simulink model "Deployed_On_CPU2"  (R2020a)
settings: Solver=ode4  StartTime=0.0  StopTime=Inf  FixedStep=0.01  RelTol=1e-3  EnableMultiTasking=on
undefined symbols (not defined in the file): C28x, CPU1, CPU2
libraries: c280xlib x47, dspobslib x27, simulink x20, c2837xDlib x1
(part 3 of 3)

== system Deployed_On_CPU2/Subsystem3/Pressure Sensor/Data acquisition/Subsystem/Delay 1ms10 ==
  function : TriggerPort  TriggerType=function-call  VariantControl=Variant
  System Outputs : Subsystem  mask(System Outputs){ShowInLibBrowser=0}
      mask prompts: ShowInLibBrowser "Simulink:masks:CustCodeMaskParam1_MP"
      settings: CopyFcn=cccopyfcn(gcb)  OpenFcn=ccopenfcn('System Outputs Function')
      mask Help: eval('feval(''rtwprivate'',''rtwhelpview'',''rtw_sys_outputs_block'')');
      mask Display: disp('System\nOutputs');

== system Deployed_On_CPU2/Subsystem3/Pressure Sensor/Data acquisition/Subsystem/Delay 1ms11 ==
  function : TriggerPort  TriggerType=function-call  VariantControl=Variant
  System Outputs : Subsystem  mask(System Outputs){ShowInLibBrowser=0}
      mask prompts: ShowInLibBrowser "Simulink:masks:CustCodeMaskParam1_MP"
      settings: CopyFcn=cccopyfcn(gcb)  OpenFcn=ccopenfcn('System Outputs Function')
      mask Help: eval('feval(''rtwprivate'',''rtwhelpview'',''rtw_sys_outputs_block'')');
      mask Display: disp('System\nOutputs');

== system Deployed_On_CPU2/Subsystem3/Pressure Sensor/Data acquisition/Subsystem/Delay 1ms12 ==
  function : TriggerPort  TriggerType=function-call  VariantControl=Variant
  System Outputs : Subsystem  mask(System Outputs){ShowInLibBrowser=0}
      mask prompts: ShowInLibBrowser "Simulink:masks:CustCodeMaskParam1_MP"
      settings: CopyFcn=cccopyfcn(gcb)  OpenFcn=ccopenfcn('System Outputs Function')
      mask Help: eval('feval(''rtwprivate'',''rtwhelpview'',''rtw_sys_outputs_block'')');
      mask Display: disp('System\nOutputs');

== system Deployed_On_CPU2/Subsystem3/Pressure Sensor/Data acquisition/Subsystem/Delay 1ms13 ==
  function : TriggerPort  TriggerType=function-call  VariantControl=Variant
  System Outputs : Subsystem  mask(System Outputs){ShowInLibBrowser=0}
      mask prompts: ShowInLibBrowser "Simulink:masks:CustCodeMaskParam1_MP"
      settings: CopyFcn=cccopyfcn(gcb)  OpenFcn=ccopenfcn('System Outputs Function')
      mask Help: eval('feval(''rtwprivate'',''rtwhelpview'',''rtw_sys_outputs_block'')');
      mask Display: disp('System\nOutputs');

== system Deployed_On_CPU2/Subsystem3/Pressure Sensor/Data acquisition/Subsystem/Delay 1ms2 ==
  function : TriggerPort  TriggerType=function-call  VariantControl=Variant
  System Outputs : Subsystem  mask(System Outputs){ShowInLibBrowser=0}
      mask prompts: ShowInLibBrowser "Simulink:masks:CustCodeMaskParam1_MP"
      settings: CopyFcn=cccopyfcn(gcb)  OpenFcn=ccopenfcn('System Outputs Function')
      mask Help: eval('feval(''rtwprivate'',''rtwhelpview'',''rtw_sys_outputs_block'')');
      mask Display: disp('System\nOutputs');

== system Deployed_On_CPU2/Subsystem3/Pressure Sensor/Data acquisition/Subsystem/Delay 1ms3 ==
  function : TriggerPort  TriggerType=function-call  VariantControl=Variant
  System Outputs : Subsystem  mask(System Outputs){ShowInLibBrowser=0}
      mask prompts: ShowInLibBrowser "Simulink:masks:CustCodeMaskParam1_MP"
      settings: CopyFcn=cccopyfcn(gcb)  OpenFcn=ccopenfcn('System Outputs Function')
      mask Help: eval('feval(''rtwprivate'',''rtwhelpview'',''rtw_sys_outputs_block'')');
      mask Display: disp('System\nOutputs');

== system Deployed_On_CPU2/Subsystem3/Pressure Sensor/Data acquisition/Subsystem/Delay 1ms4 ==
  function : TriggerPort  TriggerType=function-call  VariantControl=Variant
  System Outputs : Subsystem  mask(System Outputs){ShowInLibBrowser=0}
      mask prompts: ShowInLibBrowser "Simulink:masks:CustCodeMaskParam1_MP"
      settings: CopyFcn=cccopyfcn(gcb)  OpenFcn=ccopenfcn('System Outputs Function')
      mask Help: eval('feval(''rtwprivate'',''rtwhelpview'',''rtw_sys_outputs_block'')');
      mask Display: disp('System\nOutputs');

== system Deployed_On_CPU2/Subsystem3/Pressure Sensor/Data acquisition/Subsystem/Delay 1ms5 ==
  function : TriggerPort  TriggerType=function-call  VariantControl=Variant
  System Outputs : Subsystem  mask(System Outputs){ShowInLibBrowser=0}
      mask prompts: ShowInLibBrowser "Simulink:masks:CustCodeMaskParam1_MP"
      settings: CopyFcn=cccopyfcn(gcb)  OpenFcn=ccopenfcn('System Outputs Function')
      mask Help: eval('feval(''rtwprivate'',''rtwhelpview'',''rtw_sys_outputs_block'')');
      mask Display: disp('System\nOutputs');

== system Deployed_On_CPU2/Subsystem3/Pressure Sensor/Data acquisition/Subsystem/Delay 1ms6 ==
  function : TriggerPort  TriggerType=function-call  VariantControl=Variant
  System Outputs : Subsystem  mask(System Outputs){ShowInLibBrowser=0}
      mask prompts: ShowInLibBrowser "Simulink:masks:CustCodeMaskParam1_MP"
      settings: CopyFcn=cccopyfcn(gcb)  OpenFcn=ccopenfcn('System Outputs Function')
      mask Help: eval('feval(''rtwprivate'',''rtwhelpview'',''rtw_sys_outputs_block'')');
      mask Display: disp('System\nOutputs');

== system Deployed_On_CPU2/Subsystem3/Pressure Sensor/Data acquisition/Subsystem/Delay 1ms7 ==
  function : TriggerPort  TriggerType=function-call  VariantControl=Variant
  System Outputs : Subsystem  mask(System Outputs){ShowInLibBrowser=0}
      mask prompts: ShowInLibBrowser "Simulink:masks:CustCodeMaskParam1_MP"
      settings: CopyFcn=cccopyfcn(gcb)  OpenFcn=ccopenfcn('System Outputs Function')
      mask Help: eval('feval(''rtwprivate'',''rtwhelpview'',''rtw_sys_outputs_block'')');
      mask Display: disp('System\nOutputs');

== system Deployed_On_CPU2/Subsystem3/Pressure Sensor/Data acquisition/Subsystem/Delay 1ms8 ==
  function : TriggerPort  TriggerType=function-call  VariantControl=Variant
  System Outputs : Subsystem  mask(System Outputs){ShowInLibBrowser=0}
      mask prompts: ShowInLibBrowser "Simulink:masks:CustCodeMaskParam1_MP"
      settings: CopyFcn=cccopyfcn(gcb)  OpenFcn=ccopenfcn('System Outputs Function')
      mask Help: eval('feval(''rtwprivate'',''rtwhelpview'',''rtw_sys_outputs_block'')');
      mask Display: disp('System\nOutputs');

== system Deployed_On_CPU2/Subsystem3/Pressure Sensor/Data acquisition/Subsystem/Delay 1ms9 ==
  function : TriggerPort  TriggerType=function-call  VariantControl=Variant
  System Outputs : Subsystem  mask(System Outputs){ShowInLibBrowser=0}
      mask prompts: ShowInLibBrowser "Simulink:masks:CustCodeMaskParam1_MP"
      settings: CopyFcn=cccopyfcn(gcb)  OpenFcn=ccopenfcn('System Outputs Function')
      mask Help: eval('feval(''rtwprivate'',''rtwhelpview'',''rtw_sys_outputs_block'')');
      mask Display: disp('System\nOutputs');

== system Deployed_On_CPU2/Subsystem3/Pressure Sensor/Data acquisition/Subsystem/Read 6 bytes2 ==
  function : TriggerPort  TriggerType=function-call  VariantControl=Variant
  Add : Sum
  Data Type Conversion : DataTypeConversion  OutDataTypeStr=int16  ConvertRealWorld=Stored Integer (SI)
  Demux : Demux  Outputs=2
  Gain : Gain  Gain=256
  I2C Receive1 : c280xlib/I2C Receive  Priority=10  selectModule=I2C_A  addrFormat=7-Bit addressing  saSource=Specify via dialog  SAR=hex2dec('76')  bitCount=8  dataLength=2  initValue=0  NACK=off  STP=on  STR=on  sampleTime=-1  dataType=uint8
      settings: SourceProductBaseCode=TIC2000
  Terminator1 : Terminator
  Out1 : Outport
  wires:
  I2C Receive1/2 -> Terminator1/1
  I2C Receive1/1 -> Data Type Conversion/1
  Data Type Conversion/1 -> Demux/1
  Demux/1 -> Gain/1
  Demux/2 -> Add/2
  Gain/1 -> Add/1
  Add/1 -> Out1/1

== system Deployed_On_CPU2/Subsystem3/Pressure Sensor/Data acquisition/Subsystem/Read 6 bytes3 ==
  function : TriggerPort  TriggerType=function-call  VariantControl=Variant
  Add : Sum
  Data Type Conversion : DataTypeConversion  OutDataTypeStr=int16  ConvertRealWorld=Stored Integer (SI)
  Demux : Demux  Outputs=2
  Gain : Gain  Gain=256
  I2C Receive1 : c280xlib/I2C Receive  Priority=10  selectModule=I2C_A  addrFormat=7-Bit addressing  saSource=Specify via dialog  SAR=hex2dec('76')  bitCount=8  dataLength=2  initValue=0  NACK=off  STP=on  STR=on  sampleTime=-1  dataType=uint8
      settings: SourceProductBaseCode=TIC2000
  Terminator1 : Terminator
  Out1 : Outport
  wires:
  I2C Receive1/2 -> Terminator1/1
  I2C Receive1/1 -> Data Type Conversion/1
  Data Type Conversion/1 -> Demux/1
  Demux/1 -> Gain/1
  Add/1 -> Out1/1
  Gain/1 -> Add/1
  Demux/2 -> Add/2

== system Deployed_On_CPU2/Subsystem3/Pressure Sensor/Data acquisition/Subsystem/Read 6 bytes4 ==
  function : TriggerPort  TriggerType=function-call  VariantControl=Variant
  Add : Sum
  Data Type Conversion : DataTypeConversion  OutDataTypeStr=int16  ConvertRealWorld=Stored Integer (SI)
  Demux : Demux  Outputs=2
  Gain : Gain  Gain=256
  I2C Receive1 : c280xlib/I2C Receive  Priority=10  selectModule=I2C_A  addrFormat=7-Bit addressing  saSource=Specify via dialog  SAR=hex2dec('76')  bitCount=8  dataLength=2  initValue=0  NACK=off  STP=on  STR=on  sampleTime=-1  dataType=uint8
      settings: SourceProductBaseCode=TIC2000
  Terminator1 : Terminator
  Out1 : Outport
  wires:
  I2C Receive1/2 -> Terminator1/1
  I2C Receive1/1 -> Data Type Conversion/1
  Data Type Conversion/1 -> Demux/1
  Demux/1 -> Gain/1
  Add/1 -> Out1/1
  Gain/1 -> Add/1
  Demux/2 -> Add/2

== system Deployed_On_CPU2/Subsystem3/Pressure Sensor/Data acquisition/Subsystem/Read 6 bytes5 ==
  function : TriggerPort  TriggerType=function-call  VariantControl=Variant
  Add : Sum
  Data Type Conversion : DataTypeConversion  OutDataTypeStr=int16  ConvertRealWorld=Stored Integer (SI)
  Demux : Demux  Outputs=2
  Gain : Gain  Gain=256
  I2C Receive1 : c280xlib/I2C Receive  Priority=10  selectModule=I2C_A  addrFormat=7-Bit addressing  saSource=Specify via dialog  SAR=hex2dec('76')  bitCount=8  dataLength=2  initValue=0  NACK=off  STP=on  STR=on  sampleTime=-1  dataType=uint8
      settings: SourceProductBaseCode=TIC2000
  Terminator1 : Terminator
  Out1 : Outport
  wires:
  I2C Receive1/2 -> Terminator1/1
  I2C Receive1/1 -> Data Type Conversion/1
  Data Type Conversion/1 -> Demux/1
  Demux/1 -> Gain/1
  Add/1 -> Out1/1
  Gain/1 -> Add/1
  Demux/2 -> Add/2

== system Deployed_On_CPU2/Subsystem3/Pressure Sensor/Data acquisition/Subsystem/Read 6 bytes6 ==
  function : TriggerPort  TriggerType=function-call  VariantControl=Variant
  Add : Sum
  Data Type Conversion : DataTypeConversion  OutDataTypeStr=int16  ConvertRealWorld=Stored Integer (SI)
  Demux : Demux  Outputs=2
  Gain : Gain  Gain=256
  I2C Receive1 : c280xlib/I2C Receive  Priority=10  selectModule=I2C_A  addrFormat=7-Bit addressing  saSource=Specify via dialog  SAR=hex2dec('76')  bitCount=8  dataLength=2  initValue=0  NACK=off  STP=on  STR=on  sampleTime=-1  dataType=uint8
      settings: SourceProductBaseCode=TIC2000
  Terminator1 : Terminator
  Out3 : Outport
  wires:
  I2C Receive1/2 -> Terminator1/1
  I2C Receive1/1 -> Data Type Conversion/1
  Data Type Conversion/1 -> Demux/1
  Demux/1 -> Gain/1
  Add/1 -> Out3/1
  Gain/1 -> Add/1
  Demux/2 -> Add/2

== system Deployed_On_CPU2/Subsystem3/Pressure Sensor/Data acquisition/Subsystem/Read 6 bytes7 ==
  function : TriggerPort  TriggerType=function-call  VariantControl=Variant
  Add : Sum
  Data Type Conversion : DataTypeConversion  OutDataTypeStr=int16  ConvertRealWorld=Stored Integer (SI)
  Demux : Demux  Outputs=2
  Gain : Gain  Gain=256
  I2C Receive1 : c280xlib/I2C Receive  Priority=10  selectModule=I2C_A  addrFormat=7-Bit addressing  saSource=Specify via dialog  SAR=hex2dec('76')  bitCount=8  dataLength=2  initValue=0  NACK=off  STP=on  STR=on  sampleTime=-1  dataType=uint8
      settings: SourceProductBaseCode=TIC2000
  Terminator1 : Terminator
  Out1 : Outport
  wires:
  I2C Receive1/2 -> Terminator1/1
  I2C Receive1/1 -> Data Type Conversion/1
  Data Type Conversion/1 -> Demux/1
  Demux/1 -> Gain/1
  Add/1 -> Out1/1
  Gain/1 -> Add/1
  Demux/2 -> Add/2

== system Deployed_On_CPU2/Subsystem3/Pressure Sensor/Data acquisition/Subsystem2/Subsystem1 ==
  Constant1 : Constant  Value=2
  Constant2 : Constant  Value=23
  Power : Math  Operator=pow  SaturateOnIntegerOverflow=on
  Out1 : Outport
  wires:
  Constant2/1 -> Power/2
  Constant1/1 -> Power/1
  Power/1 -> Out1/1

== system Deployed_On_CPU2/Subsystem3/Pressure Sensor/Data acquisition/Subsystem/Delay 1ms1/System Outputs ==

== system Deployed_On_CPU2/Subsystem3/Pressure Sensor/Data acquisition/Subsystem/Delay 1ms10/System Outputs ==

== system Deployed_On_CPU2/Subsystem3/Pressure Sensor/Data acquisition/Subsystem/Delay 1ms11/System Outputs ==

== system Deployed_On_CPU2/Subsystem3/Pressure Sensor/Data acquisition/Subsystem/Delay 1ms12/System Outputs ==

== system Deployed_On_CPU2/Subsystem3/Pressure Sensor/Data acquisition/Subsystem/Delay 1ms13/System Outputs ==

== system Deployed_On_CPU2/Subsystem3/Pressure Sensor/Data acquisition/Subsystem/Delay 1ms2/System Outputs ==

== system Deployed_On_CPU2/Subsystem3/Pressure Sensor/Data acquisition/Subsystem/Delay 1ms3/System Outputs ==

== system Deployed_On_CPU2/Subsystem3/Pressure Sensor/Data acquisition/Subsystem/Delay 1ms4/System Outputs ==

== system Deployed_On_CPU2/Subsystem3/Pressure Sensor/Data acquisition/Subsystem/Delay 1ms5/System Outputs ==

== system Deployed_On_CPU2/Subsystem3/Pressure Sensor/Data acquisition/Subsystem/Delay 1ms6/System Outputs ==

== system Deployed_On_CPU2/Subsystem3/Pressure Sensor/Data acquisition/Subsystem/Delay 1ms7/System Outputs ==

== system Deployed_On_CPU2/Subsystem3/Pressure Sensor/Data acquisition/Subsystem/Delay 1ms8/System Outputs ==

== system Deployed_On_CPU2/Subsystem3/Pressure Sensor/Data acquisition/Subsystem/Delay 1ms9/System Outputs ==
